simulink model "UPQC_model"  (R2020b)
settings: Solver=FixedStepAuto  StartTime=0.0  StopTime=Tsim  FixedStep=Tsample  MaxStep=Tsample  RelTol=1e-3
values from neighbouring files (symbols this model uses):
  C_parallel_Series = zeros(1,4)    [Netzmodell_Ini_DL.m]    (also in workspace_Ini.mat = [1e-05 1e-05 1e-05 0])
  C_parallel_Shunt = zeros(1,4)    [Netzmodell_Ini_DL.m]    (also in workspace_Ini.mat = [1e-05 1e-05 1e-05 0])
  CC_Ki = 5    [Netzmodell_Ini_DL.m]    (also in workspace_Ini.mat)
  CC_Ki_geg = 5    [Netzmodell_Ini_DL.m]    (also in workspace_Ini.mat)
  CC_Kp = 10    [Netzmodell_Ini_DL.m]    (also in workspace_Ini.mat)
  CC_Kp_geg = 10    [Netzmodell_Ini_DL.m]    (also in workspace_Ini.mat)
  CC_OS =     [workspace_Ini.mat]
  Czk = Szenario.Czk*u    [Netzmodell_Ini_DL.m]    (also in workspace_Ini.mat = 0.003)
  fak_RVC = Szenario.fak_RVC    [Netzmodell_Ini_DL.m]    (also in workspace_Ini.mat = [1 1 1])
  fak_Uns = [1; 1; 1]    [Netzmodell_Ini_DL.m]    (also in workspace_Ini.mat = [1 1 1])
  Flicker_Schaltzeitpunkte_L1 = Schaltzeitpunkte(1,:)    [Netzmodell_Ini_DL.m]    (also in workspace_Ini.mat = 10.5)
  Flicker_Schaltzeitpunkte_L2 = Schaltzeitpunkte(2,:)    [Netzmodell_Ini_DL.m]    (also in workspace_Ini.mat = 10.5)
  Flicker_Schaltzeitpunkte_L3 = Schaltzeitpunkte(3,:)    [Netzmodell_Ini_DL.m]    (also in workspace_Ini.mat = 10.5)
  fs = [f_nom; f_nom; f_nom]    [Netzmodell_Ini_DL.m]    (also in workspace_Ini.mat = [50 50 50])
  fsw = Szenario.fsw*k    [Netzmodell_Ini_DL.m]    (also in workspace_Ini.mat = 20000)
  I_Basis_Ober_L1 = I_Basis_Ober(1)    [Netzmodell_Ini_DL.m]    (also in workspace_Ini.mat = 0)
  I_Basis_Ober_L2 = I_Basis_Ober(2)    [Netzmodell_Ini_DL.m]    (also in workspace_Ini.mat = 0)
  I_Basis_Ober_L3 = I_Basis_Ober(3)    [Netzmodell_Ini_DL.m]    (also in workspace_Ini.mat = 0)
  I_relativ_Ober_L1 = Szenario.I_relativ_Ober_L1    [Netzmodell_Ini_DL.m]    (also in workspace_Ini.mat = [0 100 0 100 100 0 100 100 0 0 0 0 ... (50 elements, 1x50)])
  I_relativ_Ober_L2 = Szenario.I_relativ_Ober_L2    [Netzmodell_Ini_DL.m]    (also in workspace_Ini.mat = [0 100 0 100 100 0 100 100 0 0 0 0 ... (50 elements, 1x50)])
  I_relativ_Ober_L3 = Szenario.I_relativ_Ober_L3    [Netzmodell_Ini_DL.m]    (also in workspace_Ini.mat = [0 100 0 100 100 0 100 100 0 0 0 0 ... (50 elements, 1x50)])
  L_Ausgang_Series = zeros(1,4)    [Netzmodell_Ini_DL.m]    (also in workspace_Ini.mat = [0.00093 0.00093 0.00093 0.00093])
  L_Ausgang_Shunt = zeros(1,4)    [Netzmodell_Ini_DL.m]    (also in workspace_Ini.mat = [0.00093 0.00093 0.00093 0.00093])
  L_Eingang_Series = zeros(1,4)    [Netzmodell_Ini_DL.m]    (also in workspace_Ini.mat = [0.00085 0.00085 0.00085 0.00085])
  L_Eingang_Shunt = zeros(1,4)    [Netzmodell_Ini_DL.m]    (also in workspace_Ini.mat = [0.00085 0.00085 0.00085 0.00085])
  Ls_in = 52.2*u/10    (= 5.22e-06)    [Netzmodell_Ini_DL.m]    (also in workspace_Ini.mat)
  Ltrans = Szenario.Ltrans*m    [Netzmodell_Ini_DL.m]    (also in workspace_Ini.mat = 0.000256)
  OS_off = 6    [Netzmodell_Ini_DL.m]    (also in workspace_Ini.mat)
  OS_on = 1    [Netzmodell_Ini_DL.m]    (also in workspace_Ini.mat)
  Phi_Ober_L1 = Phi_Ober(1)    [Netzmodell_Ini_DL.m]    (also in workspace_Ini.mat = 0)
  Phi_Ober_L2 = Phi_Ober(2)    [Netzmodell_Ini_DL.m]    (also in workspace_Ini.mat = -120)
  Phi_Ober_L3 = Phi_Ober(3)    [Netzmodell_Ini_DL.m]    (also in workspace_Ini.mat = 120)
  Phis = [0; -120; 120]    [Netzmodell_Ini_DL.m]    (also in workspace_Ini.mat = [0 -120 120])
  Pl_Flicker = Pl_Flicker*k    [Netzmodell_Ini_DL.m]    (also in workspace_Ini.mat = [5000 5000 5000])
  Pl_Grund = Szenario.Pl_Grund *k    [Netzmodell_Ini_DL.m]    (also in workspace_Ini.mat = [5 5 5])
  Pl_RVC = Pl_RVC*k    [Netzmodell_Ini_DL.m]    (also in workspace_Ini.mat = [10000 10000 10000])
  Pl_Uns = Pl_Uns*k    [Netzmodell_Ini_DL.m]    (also in workspace_Ini.mat = [25000 10 10])
  Ql_ind_Flicker = Ql_ind_Flicker*k    [Netzmodell_Ini_DL.m]    (also in workspace_Ini.mat = [0 0 0])
  Ql_ind_Grund = Szenario.Ql_ind_Grund*k    [Netzmodell_Ini_DL.m]    (also in workspace_Ini.mat = [0 0 0])
  Ql_ind_RVC = Szenario.Ql_ind_RVC*k    [Netzmodell_Ini_DL.m]    (also in workspace_Ini.mat = [0 0 0])
  Ql_ind_Uns = Ql_ind_Uns*k    [Netzmodell_Ini_DL.m]    (also in workspace_Ini.mat = [0 0 0])
  Ql_kap_Flicker = Ql_kap_Flicker*k    [Netzmodell_Ini_DL.m]    (also in workspace_Ini.mat = [0 0 0])
  Ql_kap_Grund = Szenario.Ql_kap_Grund*k    [Netzmodell_Ini_DL.m]    (also in workspace_Ini.mat = [0 0 0])
  Ql_kap_RVC = Szenario.Ql_kap_RVC*k    [Netzmodell_Ini_DL.m]    (also in workspace_Ini.mat = [0 0 0])
  Ql_kap_Uns = Ql_kap_Uns*k    [Netzmodell_Ini_DL.m]    (also in workspace_Ini.mat = [0 0 0])
  R_Ausgang_Series = zeros(1,4)    [Netzmodell_Ini_DL.m]    (also in workspace_Ini.mat = [0.1 0.1 0.1 0.1])
  R_Ausgang_Shunt = zeros(1,4)    [Netzmodell_Ini_DL.m]    (also in workspace_Ini.mat = [0.1 0.1 0.1 0.1])
  R_Eingang_Series = zeros(1,4)    [Netzmodell_Ini_DL.m]    (also in workspace_Ini.mat = [0.1 0.1 0.1 0.1])
  R_Eingang_Shunt = zeros(1,4)    [Netzmodell_Ini_DL.m]    (also in workspace_Ini.mat = [0.1 0.1 0.1 0.1])
  R_parallel_Series = zeros(1,4)    [Netzmodell_Ini_DL.m]    (also in workspace_Ini.mat = [13 13 13 0])
  R_parallel_Shunt = zeros(1,4)    [Netzmodell_Ini_DL.m]    (also in workspace_Ini.mat = [13 13 13 0])
  R_ZK_Belastung = 20    [Netzmodell_Ini_DL.m]    (also in workspace_Ini.mat)
  Rs_in = 5.2*m/10    (= 0.00052)    [Netzmodell_Ini_DL.m]    (also in workspace_Ini.mat)
  Rtrans = Szenario.Rtrans    [Netzmodell_Ini_DL.m]    (also in workspace_Ini.mat = 0.206)
  RVC_L1_on_off_Zeitpunkte = Szenario.RVC_L1_on_off_Zeitpunkte    [Netzmodell_Ini_DL.m]    (also in workspace_Ini.mat = [10.5 40 10 11 12 13 14 15])
  RVC_L2_on_off_Zeitpunkte = Szenario.RVC_L2_on_off_Zeitpunkte    [Netzmodell_Ini_DL.m]    (also in workspace_Ini.mat = [10.5 40 10 11 12 13 14 15])
  RVC_L3_on_off_Zeitpunkte = Szenario.RVC_L3_on_off_Zeitpunkte    [Netzmodell_Ini_DL.m]    (also in workspace_Ini.mat = [10.5 40 10 11 12 13 14 15])
  RVC_off = 20.5    [Netzmodell_Ini_DL.m]    (also in workspace_Ini.mat)
  RVC_on = 20    [Netzmodell_Ini_DL.m]    (also in workspace_Ini.mat)
  RVC_val = [0.8,0.8,0.8]    [Netzmodell_Ini_DL.m]    (also in workspace_Ini.mat = [0.8 0.8 0.8])
  strans = Szenario.strans    [Netzmodell_Ini_DL.m]    (also in workspace_Ini.mat = 0.25)
  t_breaker_series = tacts    [Netzmodell_Ini_DL.m]    (also in workspace_Ini.mat = 0.5)
  tact = Szenario.tact    [Netzmodell_Ini_DL.m]    (also in workspace_Ini.mat = 0.5)
  tact_OS_Regler = Szenario.tact_OS_Regler    [Netzmodell_Ini_DL.m]    (also in workspace_Ini.mat = 0.5)
  tact_QU = 10    [Netzmodell_Ini_DL.m]    (also in workspace_Ini.mat)
  tacts = Szenario.tacts    [Netzmodell_Ini_DL.m]    (also in workspace_Ini.mat = 0.5)
  Tsample = Szenario.Tsample    [Netzmodell_Ini_DL.m]    (also in workspace_Ini.mat = 5e-06)
  Uns_L1_on_off_Zeitpunkte = Szenario.Uns_L1_on_off_Zeitpunkte    [Netzmodell_Ini_DL.m]    (also in workspace_Ini.mat = [1 6 10 11 12 13 14 15])
  Uns_L2_on_off_Zeitpunkte = Szenario.Uns_L2_on_off_Zeitpunkte    [Netzmodell_Ini_DL.m]    (also in workspace_Ini.mat = [10 30 10 11 12 13 14 15])
  Uns_L3_on_off_Zeitpunkte = Szenario.Uns_L3_on_off_Zeitpunkte    [Netzmodell_Ini_DL.m]    (also in workspace_Ini.mat = [10 30 10 11 12 13 14 15])
  Us = [Us_Amp; Us_Amp; Us_Amp]    [Netzmodell_Ini_DL.m]    (also in workspace_Ini.mat = [326.598632371 326.598632371 326.598632371])
  Us_Amp = sqrt(2)*400/sqrt(3)    [Netzmodell_Ini_DL.m]    (also in workspace_Ini.mat = 326.598632371)
  VC_Ki_gegen = 30    [Netzmodell_Ini_DL.m]    (also in workspace_Ini.mat)
  VC_Ki_gegen_shunt = 15    [Netzmodell_Ini_DL.m]    (also in workspace_Ini.mat)
  VC_Ki_mit = 5    [Netzmodell_Ini_DL.m]    (also in workspace_Ini.mat)
  VC_Kp_gegen = 5    [workspace_Ini.mat]
  VC_Kp_gegen_shunt = 2    [Netzmodell_Ini_DL.m]    (also in workspace_Ini.mat)
  VC_Kp_mit = 10    [Netzmodell_Ini_DL.m]    (also in workspace_Ini.mat)
  VC_ZK_Ki = 5    [Netzmodell_Ini_DL.m]    (also in workspace_Ini.mat)
  VC_ZK_Kp = 0.5    [Netzmodell_Ini_DL.m]    (also in workspace_Ini.mat)
  Vielfache_Ober_L1 = Szenario.Vielfache_Ober_L1    [Netzmodell_Ini_DL.m]    (also in workspace_Ini.mat = [1 2 3 4 5 6 7 8 9 10 11 12 ... (50 elements, 1x50)])
  Vielfache_Ober_L2 = Szenario.Vielfache_Ober_L2    [Netzmodell_Ini_DL.m]    (also in workspace_Ini.mat = [1 2 3 4 5 6 7 8 9 10 11 12 ... (50 elements, 1x50)])
  Vielfache_Ober_L3 = Szenario.Vielfache_Ober_L3    [Netzmodell_Ini_DL.m]    (also in workspace_Ini.mat = [1 2 3 4 5 6 7 8 9 10 11 12 ... (50 elements, 1x50)])
  ZK_Belastung_off = 100    [Netzmodell_Ini_DL.m]    (also in workspace_Ini.mat)
  ZK_Belastung_on = 100    [Netzmodell_Ini_DL.m]    (also in workspace_Ini.mat)
  Zwischenkreisspannung = 700    [Netzmodell_Ini_DL.m]    (also in workspace_Ini.mat)
undefined symbols (not defined in the file or in its folder): LAusgang, RReiheL3
libraries: powerlib x221, powerlib_meascontrol x80, pid_lib x23, eeTransforms x4, eePwmGeneratorTwoLevel x2, dspstat3 x1
(part 4 of 16)

== system UPQC_model/Zwischenkreis_Shunt ==
  Add : Sum
  C Zwischenkreis1 : powerlib/Elements/Series RLC Branch  LConnTagsString=__new0  RConnTagsString=__new0  BranchType=C  Resistance=RReiheL3  Inductance=2.4e-3  SetiL0=off  InitialCurrent=0  Capacitance=C_Zwischenkreis*2  Setx0=off  InitialVoltage=350  Measurements=None
  C Zwischenkreis2 : powerlib/Elements/Series RLC Branch  LConnTagsString=__new0  RConnTagsString=__new0  BranchType=C  Resistance=RReiheL3  Inductance=2.4e-3  SetiL0=off  InitialCurrent=0  Capacitance=C_Zwischenkreis*2  Setx0=off  InitialVoltage=350  Measurements=None
  Ground : powerlib/Elements/Ground  Commented=on  LConnTagsString=a
  I DC 1 : powerlib/Measurements/Current Measurement  PhasorSimulation=off  OutputType=Complex  PSBequivalent=0
  I DC 2 : powerlib/Measurements/Current Measurement  PhasorSimulation=off  OutputType=Complex  PSBequivalent=0
  I DC 3 : powerlib/Measurements/Current Measurement  PhasorSimulation=off  OutputType=Complex  PSBequivalent=0
  I DC in : powerlib/Measurements/Current Measurement  PhasorSimulation=off  OutputType=Complex  PSBequivalent=0
  Series RLC Branch2 : powerlib/Elements/Series RLC Branch  LConnTagsString=__new0  RConnTagsString=__new0  BranchType=R  Resistance=40e3  Inductance=2.4e-3  SetiL0=off  InitialCurrent=0  Capacitance=C_Zwischenkreis  Setx0=off  InitialVoltage=0  Measurements=None
  Shunt_Zwischenkreise_I_Scope : Scope  NumInputPorts=4
  U DC: : powerlib/Measurements/Voltage Measurement  PhasorSimulation=off  OutputType=Complex  PSBequivalent=0
  DC+ out : PMIOPort  Side=Right
  DC- out : PMIOPort  Port=2  Side=Right
  DC+ in : PMIOPort  Port=3  Side=Left
  DC- in : PMIOPort  Port=4  Side=Left
  Neutral Connection : PMIOPort  Tag=PMCPort  Port=5  Side=Left
  U DC Zwischenkreis : Outport
  I DC Zwischenkreis out : Outport  Port=2
  I DC Zwischenkreis in : Outport  Port=3
  wires:
  U DC:/1 -> U DC Zwischenkreis/1
  I DC in/1 -> I DC Zwischenkreis out/1
  I DC 1/1 -> Add/1, I DC Zwischenkreis in/1, Shunt_Zwischenkreise_I_Scope/1
  I DC 2/1 -> Add/2, Shunt_Zwischenkreise_I_Scope/2
  Add/1 -> Shunt_Zwischenkreise_I_Scope/3
  I DC 3/1 -> Shunt_Zwischenkreise_I_Scope/4
  connections:
  C Zwischenkreis2/RConn1 -- Neutral Connection/RConn1 -- Ground/LConn1 -- C Zwischenkreis1/LConn1
  Series RLC Branch2/LConn1 -- I DC 3/RConn1
  I DC 2/LConn1 -- DC- in/RConn1
  I DC 1/LConn1 -- DC+ in/RConn1
  I DC in/RConn1 -- DC+ out/RConn1
  C Zwischenkreis1/RConn1 -- U DC:/LConn2 -- DC- out/RConn1 -- Series RLC Branch2/RConn1 -- I DC 2/RConn1
  U DC:/LConn1 -- I DC 3/LConn1 -- C Zwischenkreis2/LConn1 -- I DC 1/RConn1 -- I DC in/LConn1

== system UPQC_model/Messsignale/A ==
  Vabc : Inport
  I : Inport  Port=2
  Constant : Constant  Value=Us_Amp
  Demux : Demux  Outputs=3
  Divide{1..5} (5 alike) : Product  Inputs=*/
  Gain : Gain  Gain=100
  Gain1 : Gain  Gain=100
  Gain2 : Gain  Gain=0.001
  Mux : Mux  Inputs=2
  Mux1 : Mux  Inputs=2
  Mux2 : Mux  Inputs=3
  Power : powerlib_meascontrol/Measurements/Power  Freq=50  Vinit=[1, 0]  Iinit=[1, 0]  Ts=0
  Sequence Analyzer : powerlib_meascontrol/Measurements/Sequence Analyzer  Freq=f_nom  n=1  seq=Positive Negative Zero  InInit=[1, 0]  Ts=0
      settings: SourceProductBaseCode=PS
  +-0 normiert : Outport
  PQ : Outport  Port=2
  kU2,kU0 : Outport  Port=3
  Phase +-0 : Outport  Port=4
  wires:
  [Normierung] -> Divide3/2, Divide2/2, Divide1/2
  Divide1/1 -> Mux2/1, Divide5/2, Divide4/2  "+,A"
  Demux/1 -> Divide1/1
  I/1 -> Power/2
  Vabc/1 -> Power/1, Sequence Analyzer/1
  Divide3/1 -> Mux2/3, Divide5/1  "0,A"
  Demux/3 -> Divide3/1
  Constant/1 -> [Normierung]
  Power/2 -> Mux1/2  "Q, A"
  Demux/2 -> Divide2/1
  Divide2/1 -> Mux2/2, Divide4/1  "-,A"
  Sequence Analyzer/2 -> Phase +-0/1
  Power/1 -> Mux1/1  "P, A"
  Divide4/1 -> Gain/1  "kU2"
  Divide5/1 -> Gain1/1  "kU0"
  Sequence Analyzer/1 -> Demux/1
  Mux/1 -> kU2,kU0/1  "kU2, kU0"
  Mux1/1 -> Gain2/1  "PQ, A"
  Mux2/1 -> +-0 normiert/1  "+-0, A"
  Gain/1 -> Mux/1
  Gain1/1 -> Mux/2
  Gain2/1 -> PQ/1

== system UPQC_model/Messsignale/A1 ==
  Vabc : Inport
  I : Inport  Port=2
  Constant : Constant  Value=Us_Amp
  Demux : Demux  Outputs=3
  Divide{1..5} (5 alike) : Product  Inputs=*/
  Gain : Gain  Gain=100
  Gain1 : Gain  Gain=100
  Gain2 : Gain  Gain=0.001
  Mux : Mux  Inputs=2
  Mux1 : Mux  Inputs=2
  Mux2 : Mux  Inputs=3
  Power : powerlib_meascontrol/Measurements/Power  Freq=50  Vinit=[1, 0]  Iinit=[1, 0]  Ts=0
  Sequence Analyzer : powerlib_meascontrol/Measurements/Sequence Analyzer  Freq=f_nom  n=1  seq=Positive Negative Zero  InInit=[1, 0]  Ts=0
      settings: SourceProductBaseCode=PS
  +-0 normiert : Outport
  PQ : Outport  Port=2
  "kU2, kU0" : Outport  Port=3
  Phase +-0 : Outport  Port=4
  wires:
  [Normierung] -> Divide3/2, Divide2/2, Divide1/2
  Divide1/1 -> Mux2/1, Divide5/2, Divide4/2  "+,A"
  Demux/1 -> Divide1/1
  I/1 -> Power/2
  Vabc/1 -> Power/1, Sequence Analyzer/1
  Divide3/1 -> Mux2/3, Divide5/1  "0,A"
  Demux/3 -> Divide3/1
  Constant/1 -> [Normierung]
  Power/2 -> Mux1/2  "Q, A"
  Demux/2 -> Divide2/1
  Divide2/1 -> Mux2/2, Divide4/1  "-,A"
  Sequence Analyzer/2 -> Phase +-0/1
  Power/1 -> Mux1/1  "P, A"
  Divide4/1 -> Gain/1  "kU2"
  Divide5/1 -> Gain1/1  "kU0"
  Sequence Analyzer/1 -> Demux/1
  Mux/1 -> "kU2, kU0"/1  "kU2, kU0"
  Mux1/1 -> Gain2/1  "PQ, A"
  Mux2/1 -> +-0 normiert/1  "+-0, A"
  Gain/1 -> Mux/1
  Gain1/1 -> Mux/2
  Gain2/1 -> PQ/1

== system UPQC_model/Messsignale/Bneu ==
  Vabc : Inport
  I : Inport  Port=2
  Constant : Constant  Value=Us_Amp
  Demux : Demux  Outputs=3
  Divide{1..5} (5 alike) : Product  Inputs=*/
  Gain : Gain  Gain=100
  Gain1 : Gain  Gain=100
  Gain2 : Gain  Gain=0.001
  Mux : Mux  Inputs=2
  Mux1 : Mux  Inputs=2
  Mux2 : Mux  Inputs=3
  Power : powerlib_meascontrol/Measurements/Power  Freq=50  Vinit=[1, 0]  Iinit=[1, 0]  Ts=0
  Sequence Analyzer : powerlib_meascontrol/Measurements/Sequence Analyzer  Freq=f_nom  n=1  seq=Positive Negative Zero  InInit=[1, 0]  Ts=0
      settings: SourceProductBaseCode=PS
  +-0 normiert : Outport
  PQ : Outport  Port=2
  "kU2, kU0" : Outport  Port=3
  Phase +-0 : Outport  Port=4
  wires:
  [Normierung] -> Divide3/2, Divide2/2, Divide1/2
  Divide1/1 -> Mux2/1, Divide5/2, Divide4/2  "+,A"
  Demux/1 -> Divide1/1
  I/1 -> Power/2
  Vabc/1 -> Power/1, Sequence Analyzer/1
  Divide3/1 -> Mux2/3, Divide5/1  "0,A"
  Demux/3 -> Divide3/1
  Constant/1 -> [Normierung]
  Power/2 -> Mux1/2  "Q, A"
  Demux/2 -> Divide2/1
  Divide2/1 -> Mux2/2, Divide4/1  "-,A"
  Sequence Analyzer/2 -> Phase +-0/1
  Power/1 -> Mux1/1  "P, A"
  Divide4/1 -> Gain/1  "kU2"
  Divide5/1 -> Gain1/1  "kU0"
  Sequence Analyzer/1 -> Demux/1
  Mux/1 -> "kU2, kU0"/1  "kU2, kU0"
  Mux1/1 -> Gain2/1  "PQ, A"
  Mux2/1 -> +-0 normiert/1  "+-0, A"
  Gain/1 -> Mux/1
  Gain1/1 -> Mux/2
  Gain2/1 -> PQ/1

== system UPQC_model/Oberschwingung Last/50 Times Input ==
  Constant : Constant  Value=0
  Mux : Mux  Inputs=50
  Out1 : Outport
  wires:
  Mux/1 -> Out1/1
  Constant/1 -> Mux/50, Mux/49, Mux/48, Mux/47, Mux/46, Mux/45, Mux/44, Mux/43, Mux/42, Mux/41, Mux/40, Mux/39, Mux/38, Mux/37, Mux/36, Mux/35, Mux/34, Mux/33, Mux/32, Mux/31, Mux/30, Mux/29, Mux/28, Mux/27, Mux/26, Mux/25, Mux/24, Mux/23, Mux/22, Mux/21, Mux/20, Mux/19, Mux/18, Mux/17, Mux/16, Mux/15, Mux/14, Mux/13, Mux/12, Mux/11, Mux/10, Mux/9, Mux/8, Mux/7, Mux/6, Mux/5, Mux/4, Mux/3, Mux/2, Mux/1

== system UPQC_model/Oberschwingung Last/Subsystem1 ==
  Constant : Constant  Value=-120
  Mux : Mux  Inputs=50
  Out1 : Outport
  wires:
  Mux/1 -> Out1/1
  Constant/1 -> Mux/50, Mux/49, Mux/48, Mux/47, Mux/46, Mux/45, Mux/44, Mux/43, Mux/42, Mux/41, Mux/40, Mux/39, Mux/38, Mux/37, Mux/36, Mux/35, Mux/34, Mux/33, Mux/32, Mux/31, Mux/30, Mux/29, Mux/28, Mux/27, Mux/26, Mux/25, Mux/24, Mux/23, Mux/22, Mux/21, Mux/20, Mux/19, Mux/18, Mux/17, Mux/16, Mux/15, Mux/14, Mux/13, Mux/12, Mux/11, Mux/10, Mux/9, Mux/8, Mux/7, Mux/6, Mux/5, Mux/4, Mux/3, Mux/2, Mux/1

== system UPQC_model/Oberschwingung Last/Subsystem2 ==
  Constant : Constant  Value=120
  Mux : Mux  Inputs=50
  Out1 : Outport
  wires:
  Constant/1 -> Mux/1, Mux/2, Mux/3, Mux/4, Mux/5, Mux/6, Mux/7, Mux/8, Mux/9, Mux/10, Mux/11, Mux/12, Mux/13, Mux/14, Mux/15, Mux/16, Mux/17, Mux/18, Mux/19, Mux/20, Mux/21, Mux/22, Mux/23, Mux/24, Mux/25, Mux/26, Mux/27, Mux/28, Mux/29, Mux/30, Mux/31, Mux/32, Mux/33, Mux/34, Mux/35, Mux/36, Mux/37, Mux/38, Mux/39, Mux/40, Mux/41, Mux/42, Mux/43, Mux/44, Mux/45, Mux/46, Mux/47, Mux/48, Mux/49, Mux/50
  Mux/1 -> Out1/1

== system UPQC_model/Series UPQC/Serienkompensator ==
  note: OUTPUT
  note: INPUT
  note: --------------------------------------------------------------------------------
  note: --------------------------------------------------------------------------------
  note: --------------------------------------------------------------------------------
  note: --------------------------------------------------------------------------------
  note: SETPOINT GENERATION
  note: ARCHIV
  note: SPANNUNGSREGELUNG
  note: REFERENZSPANNUNG LAST
  note: ISTSPANNUNG LAST
  enable : Inport
  PLL : Inport  Port=2
  VSC-Strom : Inport  Port=3
  PCC-Spg : Inport  Port=4
  Bus Selector : BusSelector  OutputSignals=phipll
  Bus Selector1 : BusSelector  OutputSignals=udqp1_f,udqg1_f
  Gegensystem : Subsystem
  Mitsystem : Subsystem
  Setpoints Series : Scope  NumInputPorts=2
  Step : Step  Time=tacts  SampleTime=0
  Subsystem : Subsystem
  Subsystem3 : Subsystem
  Subsystem5 : Subsystem
  Udq_Series_C : Subsystem
  dq+ Soll VSC Series : Scope
  dq- Last : Scope
  dq- Soll VSC Series : Scope
  sp : Outport
  wires:
  PCC-Spg/1 -> [ext_spg]
  VSC-Strom/1 -> [int_strom]
  [setpoints] -> sp/1
  enable/1 -> [enable]
  [ext_spg] -> Setpoints Series/1  "C_Netzspannung_abc"
  [udq0gegREF] -> Gegensystem/1(udq0ref)
  [udq0geg] -> Gegensystem/2(udq0)
  [phipll] -> Subsystem3/2(phiPLL)
  Subsystem3/1(sp) -> [setpoints], Setpoints Series/2  "Setpoints_Series"
  Subsystem/1(udq0ref) -> [udq0mitREF]
  Subsystem5/1(udq0ref) -> [udq0gegREF]
  PLL/1 -> Bus Selector/1
  Bus Selector/1 -> [phipll]  "<phipll>"
  [udq0mitREF] -> Mitsystem/1(udq0ref)
  [udq0mit] -> Mitsystem/2(udq0)
  Step/1 -> Mitsystem/Enable, Gegensystem/Enable
  [udq0mitsp] -> Subsystem3/1(upos)
  Mitsystem/1(udq0*) -> dq+ Soll VSC Series/1, [udq0mitsp]  "udq0*+"
  Gegensystem/1(udq0*) -> dq- Soll VSC Series/1, [udq0gegsp]  "udq0*-"
  [phipll] -> Udq_Series_C/2(In1)  "pll"
  Udq_Series_C/1(Out5) -> Bus Selector1/1
  Bus Selector1/1 -> [udq0mit]  "<udqp1_f>"
  Bus Selector1/2 -> dq- Last/1, [udq0geg]  "<udqg1_f>"
  [ext_spg] -> Udq_Series_C/1(In2)
  [udq0gegsp] -> Subsystem3/3(uneg)

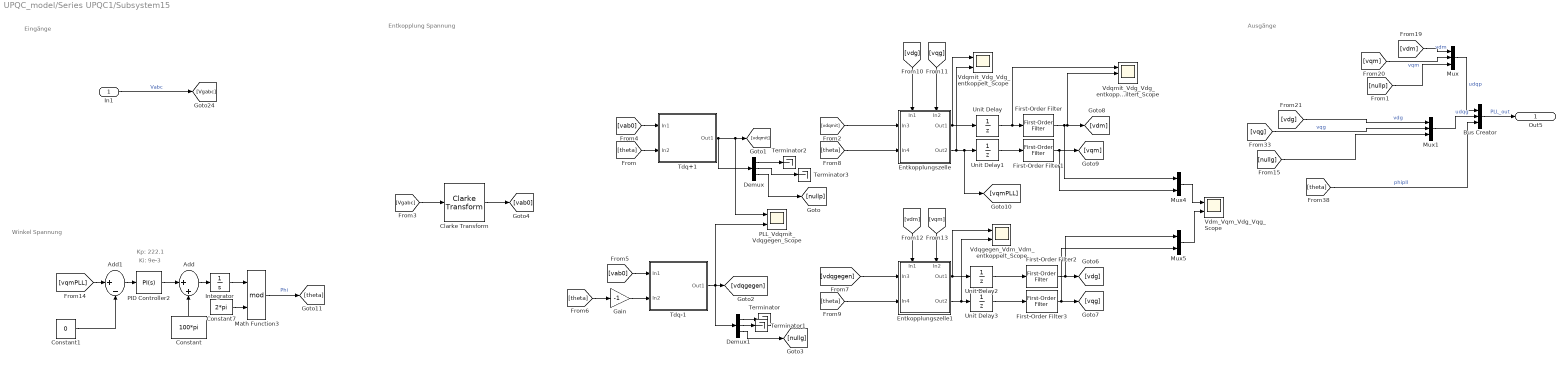
== system UPQC_model/Series UPQC1/Subsystem15 ==
  note: Ki: 9e-3
  note: Kp: 222.1
  note: Winkel Spannung
  note: Ausgänge
  note: Eingänge
  note: Entkopplung Spannung
  In1 : Inport
  Add : Sum  Inputs=|++
  Add1 : Sum  Inputs=|+-
  Bus Creator : BusCreator  Inputs=3
  Clarke Transform : eeTransforms/Clarke Transform  PowerInvariant=off
      settings: SourceProductBaseCode=PS
  Constant : Constant  Value=100*pi
  Constant1 : Constant  Value=0
  Constant7 : Constant  Value=2*pi
  Demux : Demux  Outputs=3
  Demux1 : Demux  Outputs=3
  Entkopplungszelle : Subsystem
      settings: PortSchema="{\"entries\":[{\"content\":{\"sides\":[{\"content\":{\"connectorIds\":[\"In1\",\"In2\"]},\"type\":\"ConnectorPlacement.EquallySpacedRectSide\",\"uuid\":\"e8e24803-2fc0-483c-82f9-6ee33f65ebd9\"},{\"content\":{\"connectorIds\":[\"Out1\",\"Out2\"],\"side\":\"RIGHT\"},\"type\":\"ConnectorPlacement.EquallySpacedRectSide\",\"uuid\":\"e11e5831-ab5e-42bb-bd0b-63825273f403\"},{\"content\":{\"connectorIds\":[\"In3\",\"In4\"],\"side\":\"TOP\"},\"type\":\"ConnectorPlacement.EquallySpacedRectSide\",\"uuid\":\"2b39bd07-2b6e-4e89-bb54-1321cea2c793\"},{\"content\":{\"connectorIds\":[],\"side\":\"HIDDEN\"},\"type\":\"ConnectorPlacement.EquallySpacedRectSide\",\"uuid\":\"a99c5943-5af0-4d11-8875-695bd24f17f4\"}]},\"type\":\"ConnectorPlacement.EquallySpacedConnector\",\"uuid\":\"a2a714db-f067-4e0e-8919-f68d1dab84ba\"}],\"packageUris\":[\"http://schema.mathworks.com/mf0/Connector/R2020b\"],\"version\":\"1.0\"}"
  Entkopplungszelle1 : Subsystem
      settings: PortSchema="{\"entries\":[{\"content\":{\"sides\":[{\"content\":{\"connectorIds\":[\"In1\",\"In2\"]},\"type\":\"ConnectorPlacement.EquallySpacedRectSide\",\"uuid\":\"e8e24803-2fc0-483c-82f9-6ee33f65ebd9\"},{\"content\":{\"connectorIds\":[\"Out1\",\"Out2\"],\"side\":\"RIGHT\"},\"type\":\"ConnectorPlacement.EquallySpacedRectSide\",\"uuid\":\"e11e5831-ab5e-42bb-bd0b-63825273f403\"},{\"content\":{\"connectorIds\":[\"In3\",\"In4\"],\"side\":\"TOP\"},\"type\":\"ConnectorPlacement.EquallySpacedRectSide\",\"uuid\":\"2b39bd07-2b6e-4e89-bb54-1321cea2c793\"},{\"content\":{\"connectorIds\":[],\"side\":\"HIDDEN\"},\"type\":\"ConnectorPlacement.EquallySpacedRectSide\",\"uuid\":\"a99c5943-5af0-4d11-8875-695bd24f17f4\"}]},\"type\":\"ConnectorPlacement.EquallySpacedConnector\",\"uuid\":\"a2a714db-f067-4e0e-8919-f68d1dab84ba\"}],\"packageUris\":[\"http://schema.mathworks.com/mf0/Connector/R2020b\"],\"version\":\"1.0\"}"
  First-Order Filter{,1..3} (4 alike) : powerlib_meascontrol/Filters/First-Order Filter  FilterType=Lowpass  Tc=1/(2*pi*50/sqrt(2))  Ts=0  Initialize=off  Vac_Init=[0, 0, 60]  Vdc_Init=0  PlotResponse=off  FreqRange="[0,  30,  1]"
  Gain : Gain  Gain=-1
  Integrator : Integrator
  Math Function3 : Math  Operator=mod  SignedPower=on  SaturateOnIntegerOverflow=on
  Mux : Mux  Inputs=3
  Mux1 : Mux  Inputs=3
  Mux4 : Mux  Inputs=2
  Mux5 : Mux  Inputs=2
  PID Controller2 : pid_lib/PID Controller  Controller=PI  Form=Parallel  TimeDomain=Continuous-time  UseExternalTs=off  SampleTime=-1  IntegratorMethod=Forward Euler  FilterMethod=Forward Euler  ControllerParametersSource=internal  P=222.1  I=9e-3  D=0  UseFilter=on  N=100  TunerSelectOption=Transfer Function Based (PID Tuner App)  InitialConditionSource=internal  InitialConditionForIntegrator=0  InitialConditionForFilter=0  DifferentiatorICPrevScaledInput=0  ExternalReset=none  TrackingMode=off  Kt=1  LimitOutput=off  SatLimitsSource=internal  UpperSaturationLimit=inf  LowerSaturationLimit=-inf  LinearizeAsGain=on  AntiWindupMode=none  Kb=1  POutMin=[]  POutMax=[]  IOutMin=[]  IOutMax=[]  DOutMin=[]  DOutMax=[]  NOutMin=[]  NOutMax=[]  SumOutMin=[]  SumOutMax=[]  SaturationOutMin=[]  SaturationOutMax=[]  PParamMin=[]  PParamMax=[]  IParamMin=[]  IParamMax=[]  DParamMin=[]  DParamMax=[]  NParamMin=[]  NParamMax=[]  KbParamMin=[]  KbParamMax=[]  KtParamMin=[]  KtParamMax=[]  KbOutMin=[]  KbOutMax=[]  KtOutMin=[]  KtOutMax=[]  IntegratorOutMin=[]  IntegratorOutMax=[]  FilterOutMin=[]  FilterOutMax=[]  SumI1OutMin=[]  SumI1OutMax=[]  SumI2OutMin=[]  SumI2OutMax=[]  SumI3OutMin=[]  SumI3OutMax=[]  SumI4OutMin=[]  SumI4OutMax=[]  SumDOutMin=[]  SumDOutMax=[]  DifferentiatorOutMin=[]  DifferentiatorOutMax=[]  FilterDiffOutCoefMin=[]  FilterDiffOutCoefMax=[]  ReciprocalOutMin=[]  ReciprocalOutMax=[]  SumDenOutMin=[]  SumDenOutMax=[]  SumNumOutMin=[]  SumNumOutMax=[]  DivideOutMin=[]  DivideOutMax=[]  UdiffTsProdOutMin=[]  UdiffTsProdOutMax=[]  NTsProdOutMin=[]  NTsProdOutMax=[]  UintegralTsProdOutMin=[]  UintegralTsProdOutMax=[]  UngainTsProdOutMin=[]  UngainTsProdOutMax=[]  IntegratorContinuousStateAttributes=''  IntegratorStateMustResolveToSignalObject=off  IntegratorRTWStateStorageClass=Auto  FilterContinuousStateAttributes=''  FilterStateMustResolveToSignalObject=off  FilterRTWStateStorageClass=Auto  ParallelPVariant=InternalParameters  IdealPVariant=Disabled  IVariant=InternalParameters  DVariant=Disabled  IntegratorVariant=Continuous  SatVariant=Disabled  AWVariant=Passthrough  PCopyVariant=Disabled  TRVariant=Disabled  FdbkBlocksVariant=Forward  IdealPFdbkVariant=Disabled  SatFdbkVariant=Disabled  DerivativeFilterVariant=Disabled  NVariant=Disabled  NCopyVariant=Disabled_SignalSpec  FilterICVariant=Disabled  IntegratorICVariant=InternalICs  ExternalResetVariant=Disabled  TRSumVariant=Passthrough  SumFdbkVariant=Disabled  SumVariant=Sum_PI  TsampFilterVariant=InternalTs  TsampNgainVariant=Passthrough  TsampIntegralVariant=Passthrough  ExternalSaturationOutDataTypeStr=Inherit: Same as second input
  PLL_Vdqmit_Vdqgegen_Scope : Scope  NumInputPorts=2
  Tdq+1 : Subsystem
  Tdq-1 : Subsystem
  Terminator{,1..3} (4 alike) : Terminator
  Unit Delay{,1..3} (4 alike) : UnitDelay  SampleTime=-1  HasFrameUpgradeWarning=on
  Vdm_Vqm_Vdg_Vqg_Scope : Scope  NumInputPorts=2
  Vdqgegen_Vdm_Vdm_entkoppelt_Scope : Scope  NumInputPorts=2
  Vdqmit_Vdg_Vdg_entkoppelt_Scope : Scope  NumInputPorts=2
  Vdqmit_Vdg_Vdg_entkoppelt_gefiltert_Scope : Scope  NumInputPorts=3
  Out5 : Outport
  wires:
  [theta] -> Entkopplungszelle/2(In4)
  Clarke Transform/1 -> [vab0]
  [vdqmit] -> Entkopplungszelle/1(In3)
  [vqm] -> Entkopplungszelle1/4(In2)
  Entkopplungszelle1/2(Out2) -> Vdqgegen_Vdm_Vdm_entkoppelt_Scope/2, Unit Delay3/1
  Constant/1 -> Add/2
  Tdq-1/1(Out1) -> Demux1/1, [vdqgegen], PLL_Vdqmit_Vdqgegen_Scope/2
  [vdg] -> Entkopplungszelle/3(In1)
  Unit Delay/1 -> Vdqmit_Vdg_Vdg_entkoppelt_gefiltert_Scope/1, First-Order Filter/1
  Entkopplungszelle/2(Out2) -> Vdqmit_Vdg_Vdg_entkoppelt_Scope/2, [vqmPLL], Unit Delay1/1
  Constant1/1 -> Add1/2
  [vqmPLL] -> Add1/1
  Integrator/1 -> Math Function3/1
  [theta] -> Gain/1
  Gain/1 -> Tdq-1/2(In2)
  [vdm] -> Entkopplungszelle1/3(In1)
  [vqg] -> Entkopplungszelle/4(In2)
  Add/1 -> Integrator/1
  Unit Delay3/1 -> First-Order Filter3/1
  First-Order Filter/1 -> Mux4/1, [vdm], Vdqmit_Vdg_Vdg_entkoppelt_gefiltert_Scope/2
  [theta] -> Tdq+1/2(In2)
  Constant7/1 -> Math Function3/2
  [vab0] -> Tdq-1/1(In1)
  PID Controller2/1 -> Add/1
  Unit Delay1/1 -> First-Order Filter1/1
  Add1/1 -> PID Controller2/1
  [theta] -> Entkopplungszelle1/2(In4)
  [vdqgegen] -> Entkopplungszelle1/1(In3)
  In1/1 -> [Vgabc]  "Vabc"
  [vdg] -> Mux1/1  "vdg"
  [vqg] -> Mux1/2  "vqg"
  [theta] -> Bus Creator/3  "phipll"
  Math Function3/1 -> [theta]  "Phi"
  [vab0] -> Tdq+1/1(In1)
  Entkopplungszelle/1(Out1) -> Vdqmit_Vdg_Vdg_entkoppelt_Scope/1, Unit Delay/1
  Entkopplungszelle1/1(Out1) -> Vdqgegen_Vdm_Vdm_entkoppelt_Scope/1, Unit Delay2/1
  [Vgabc] -> Clarke Transform/1
  Bus Creator/1 -> Out5/1  "PLL_out"
  Tdq+1/1(Out1) -> Demux/1, PLL_Vdqmit_Vdqgegen_Scope/1, [vdqmit]
  Demux1/1 -> Terminator/1
  Demux1/2 -> Terminator1/1
  Demux/1 -> Terminator2/1
  Demux/2 -> Terminator3/1
  Demux/3 -> [nullp]
  Demux1/3 -> [nullg]
  [vdm] -> Mux/1  "vdm"
  [vqm] -> Mux/2  "vqm"
  [nullp] -> Mux/3
  Mux/1 -> Bus Creator/1  "udqp"
  [nullg] -> Mux1/3
  Mux1/1 -> Bus Creator/2  "udqg"
  Unit Delay2/1 -> First-Order Filter2/1
  Mux5/1 -> Vdm_Vqm_Vdg_Vqg_Scope/2
  Mux4/1 -> Vdm_Vqm_Vdg_Vqg_Scope/1
  First-Order Filter1/1 -> [vqm], Mux4/2
  First-Order Filter2/1 -> [vdg], Mux5/1
  First-Order Filter3/1 -> [vqg], Mux5/2

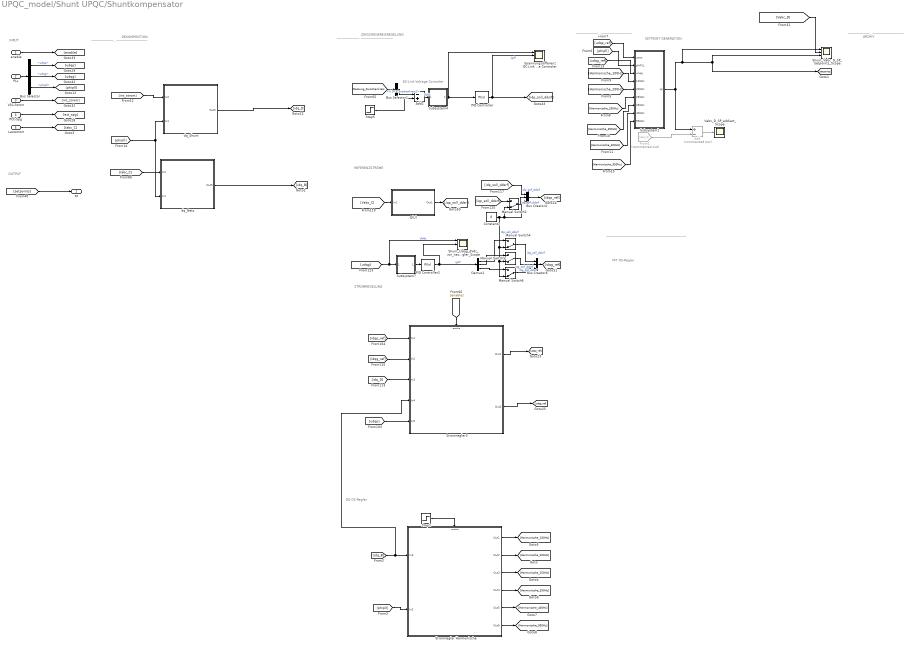
== system UPQC_model/Shunt UPQC/Shuntkompensator ==
  note: DC-Link Voltage Controler
  note: --------------------------------------------------------------------------------
  note: DEKOMPOSITION
  note: REFERENZSTRÖME
  note: STROMREGELUNG
  note: ARCHIV
  note: OUTPUT
  note: INPUT
  note: SETPOINT GENERATION
  note: --------------------------------------------------------------------------------
  note: --------------------------------------------------------------------------------
  note: --------------------------------------------------------------------------------
  note: --------------------------------------------------------------------------------
  note: FFT OS-Regler
  note: DQ OS-Regler
  note: ZWISCHENKREISREGELUNG
  enable : Inport
  PLL : Inport  Port=2
  VSC-Strom : Inport  Port=3
  PCC-Spg : Inport  Port=4
  Laststrom : Inport  Port=5
  Add : Sum  Commented=on  Inputs=+-
  Add2 : Sum  Inputs=-+
  Bus Creator4 : BusCreator  Inputs=3
  Bus Creator6 : BusCreator  Inputs=3
  Bus Selector : BusSelector  OutputSignals=udqp,udqg,phipll
  Bus Selector1 : BusSelector  OutputSignals=U DC Zwischenkreis1
  Constant1 : Constant  Value=0
  Demux1 : Demux  Outputs=3
  From1 : From  Commented=on  GotoTag=Vabc_D  TagVisibility=global
  Manual Switch{2,4..6} (4 alike) : ManualSwitch  CurrentSetting=0
  PID Controller : pid_lib/PID Controller  Controller=PI  Form=Parallel  TimeDomain=Continuous-time  UseExternalTs=off  SampleTime=-1  IntegratorMethod=Forward Euler  FilterMethod=Forward Euler  ControllerParametersSource=internal  P=VC_ZK_Kp  I=VC_ZK_Ki  D=0  UseFilter=on  N=100  TunerSelectOption=Transfer Function Based (PID Tuner App)  InitialConditionSource=internal  InitialConditionForIntegrator=0  InitialConditionForFilter=0  DifferentiatorICPrevScaledInput=0  ExternalReset=none  TrackingMode=off  Kt=1  LimitOutput=off  SatLimitsSource=internal  UpperSaturationLimit=5  LowerSaturationLimit=-5  LinearizeAsGain=on  AntiWindupMode=none  Kb=1  POutMin=[]  POutMax=[]  IOutMin=[]  IOutMax=[]  DOutMin=[]  DOutMax=[]  NOutMin=[]  NOutMax=[]  SumOutMin=[]  SumOutMax=[]  SaturationOutMin=[]  SaturationOutMax=[]  PParamMin=[]  PParamMax=[]  IParamMin=[]  IParamMax=[]  DParamMin=[]  DParamMax=[]  NParamMin=[]  NParamMax=[]  KbParamMin=[]  KbParamMax=[]  KtParamMin=[]  KtParamMax=[]  KbOutMin=[]  KbOutMax=[]  KtOutMin=[]  KtOutMax=[]  IntegratorOutMin=[]  IntegratorOutMax=[]  FilterOutMin=[]  FilterOutMax=[]  SumI1OutMin=[]  SumI1OutMax=[]  SumI2OutMin=[]  SumI2OutMax=[]  SumI3OutMin=[]  SumI3OutMax=[]  SumI4OutMin=[]  SumI4OutMax=[]  SumDOutMin=[]  SumDOutMax=[]  DifferentiatorOutMin=[]  DifferentiatorOutMax=[]  FilterDiffOutCoefMin=[]  FilterDiffOutCoefMax=[]  ReciprocalOutMin=[]  ReciprocalOutMax=[]  SumDenOutMin=[]  SumDenOutMax=[]  SumNumOutMin=[]  SumNumOutMax=[]  DivideOutMin=[]  DivideOutMax=[]  UdiffTsProdOutMin=[]  UdiffTsProdOutMax=[]  NTsProdOutMin=[]  NTsProdOutMax=[]  UintegralTsProdOutMin=[]  UintegralTsProdOutMax=[]  UngainTsProdOutMin=[]  UngainTsProdOutMax=[]  IntegratorContinuousStateAttributes=''  IntegratorStateMustResolveToSignalObject=off  IntegratorRTWStateStorageClass=Auto  FilterContinuousStateAttributes=''  FilterStateMustResolveToSignalObject=off  FilterRTWStateStorageClass=Auto  ParallelPVariant=InternalParameters  IdealPVariant=Disabled  IVariant=InternalParameters  DVariant=Disabled  IntegratorVariant=Continuous  SatVariant=Disabled  AWVariant=Passthrough  PCopyVariant=Disabled  TRVariant=Disabled  FdbkBlocksVariant=Forward  IdealPFdbkVariant=Disabled  SatFdbkVariant=Disabled  DerivativeFilterVariant=Disabled  NVariant=Disabled  NCopyVariant=Disabled_SignalSpec  FilterICVariant=Disabled  IntegratorICVariant=InternalICs  ExternalResetVariant=Disabled  TRSumVariant=Passthrough  SumFdbkVariant=Disabled  SumVariant=Sum_PI  TsampFilterVariant=InternalTs  TsampNgainVariant=Passthrough  TsampIntegralVariant=Passthrough  ExternalSaturationOutDataTypeStr=Inherit: Same as second input
  PID Controller2 : pid_lib/PID Controller  Controller=PI  Form=Parallel  TimeDomain=Continuous-time  UseExternalTs=off  SampleTime=-1  IntegratorMethod=Forward Euler  FilterMethod=Forward Euler  ControllerParametersSource=internal  P=VC_Kp_gegen_shunt  I=VC_Ki_gegen_shunt  D=0  UseFilter=on  N=100  TunerSelectOption=Transfer Function Based (PID Tuner App)  InitialConditionSource=internal  InitialConditionForIntegrator=0  InitialConditionForFilter=0  DifferentiatorICPrevScaledInput=0  ExternalReset=none  TrackingMode=off  Kt=1  LimitOutput=off  SatLimitsSource=internal  UpperSaturationLimit=5  LowerSaturationLimit=-5  LinearizeAsGain=on  AntiWindupMode=none  Kb=1  POutMin=[]  POutMax=[]  IOutMin=[]  IOutMax=[]  DOutMin=[]  DOutMax=[]  NOutMin=[]  NOutMax=[]  SumOutMin=[]  SumOutMax=[]  SaturationOutMin=[]  SaturationOutMax=[]  PParamMin=[]  PParamMax=[]  IParamMin=[]  IParamMax=[]  DParamMin=[]  DParamMax=[]  NParamMin=[]  NParamMax=[]  KbParamMin=[]  KbParamMax=[]  KtParamMin=[]  KtParamMax=[]  KbOutMin=[]  KbOutMax=[]  KtOutMin=[]  KtOutMax=[]  IntegratorOutMin=[]  IntegratorOutMax=[]  FilterOutMin=[]  FilterOutMax=[]  SumI1OutMin=[]  SumI1OutMax=[]  SumI2OutMin=[]  SumI2OutMax=[]  SumI3OutMin=[]  SumI3OutMax=[]  SumI4OutMin=[]  SumI4OutMax=[]  SumDOutMin=[]  SumDOutMax=[]  DifferentiatorOutMin=[]  DifferentiatorOutMax=[]  FilterDiffOutCoefMin=[]  FilterDiffOutCoefMax=[]  ReciprocalOutMin=[]  ReciprocalOutMax=[]  SumDenOutMin=[]  SumDenOutMax=[]  SumNumOutMin=[]  SumNumOutMax=[]  DivideOutMin=[]  DivideOutMax=[]  UdiffTsProdOutMin=[]  UdiffTsProdOutMax=[]  NTsProdOutMin=[]  NTsProdOutMax=[]  UintegralTsProdOutMin=[]  UintegralTsProdOutMax=[]  UngainTsProdOutMin=[]  UngainTsProdOutMax=[]  IntegratorContinuousStateAttributes=''  IntegratorStateMustResolveToSignalObject=off  IntegratorRTWStateStorageClass=Auto  FilterContinuousStateAttributes=''  FilterStateMustResolveToSignalObject=off  FilterRTWStateStorageClass=Auto  ParallelPVariant=InternalParameters  IdealPVariant=Disabled  IVariant=InternalParameters  DVariant=Disabled  IntegratorVariant=Continuous  SatVariant=Disabled  AWVariant=Passthrough  PCopyVariant=Disabled  TRVariant=Disabled  FdbkBlocksVariant=Forward  IdealPFdbkVariant=Disabled  SatFdbkVariant=Disabled  DerivativeFilterVariant=Disabled  NVariant=Disabled  NCopyVariant=Disabled_SignalSpec  FilterICVariant=Disabled  IntegratorICVariant=InternalICs  ExternalResetVariant=Disabled  TRSumVariant=Passthrough  SumFdbkVariant=Disabled  SumVariant=Sum_PI  TsampFilterVariant=InternalTs  TsampNgainVariant=Passthrough  TsampIntegralVariant=Passthrough  ExternalSaturationOutDataTypeStr=Inherit: Same as second input
  Q(U) : Subsystem
  Shunt_Udqg_dVdc_vor_nach_PIRegler_Scope : Scope  NumInputPorts=3
  Shunt_Vabc_D_SP_Setpoints_Scope : Scope  NumInputPorts=3
  Spannungsdifferenz DC Link Voltage Controler : Scope  NumInputPorts=3
  Step1 : Step  Time=tact_OS_Regler  SampleTime=0
  Step5 : Step  Time=100  Before=Zwischenkreisspannung  After=Zwischenkreisspannung+0  SampleTime=0
  Stromregler Harmonische : Subsystem
  Stromregler3 : Subsystem
  Subsystem1 : Subsystem
  Subsystem4 : Subsystem
  Subsystem7 : Subsystem
  Vabc_D_SP_addiert_Scope : Scope
  dq_Netz : Subsystem
  dq_Shunt : Subsystem
  sp : Outport
  wires:
  [int_strom] -> dq_Shunt/1(In2)
  enable/1 -> [enable]
  [setpoints] -> sp/1
  PCC-Spg/1 -> [ext_spg]
  Laststrom/1 -> [Iabc_C]
  VSC-Strom/1 -> [int_strom]
  PLL/1 -> Bus Selector/1
  [phipll] -> dq_Netz/2(In1), dq_Shunt/2(In1)
  [Iabc_C] -> dq_Netz/1(In2)
  Bus Selector/1 -> [udqp]  "<udqp>"
  Bus Selector/2 -> [udqg]  "<udqg>"
  Subsystem1/1(sp) -> Add/1, Shunt_Vabc_D_SP_Setpoints_Scope/3, [setpoints], Shunt_Vabc_D_SP_Setpoints_Scope/1
  [Messung_Zwischenkreis] -> Bus Selector1/1
  Bus Selector1/1 -> Add2/1  "<U DC Zwischenkreis1>"
  PID Controller/1 -> Spannungsdifferenz DC Link Voltage Controler/2, [idp_soll_ddsrf]  "igd*"
  Step5/1 -> Add2/2
  Stromregler3/2(Out2) -> [udqg_ref]
  Stromregler3/1(Out1) -> [udqp_ref]
  [enable] -> Stromregler3/Enable
  [idqp_ref] -> Stromregler3/1(In1)
  [idqg_ref] -> Stromregler3/2(In2)
  Bus Creator4/1 -> [idqp_ref]
  [idp_soll_ddsrf] -> Bus Creator4/1  "idp_soll_ddsrf"
  [idq_D] -> Stromregler3/3(In3)
  [Vabc_C] -> Q(U)/1(In1)
  Q(U)/1(Out1) -> [iqp_soll_ddsrf]
  Add2/1 -> Subsystem4/1(dVdc)  "dVdc"
  [udqg] -> Shunt_Udqg_dVdc_vor_nach_PIRegler_Scope/1, Subsystem7/1(dVdc)  "dVdc"
  PID Controller2/1 -> Demux1/1, Shunt_Udqg_dVdc_vor_nach_PIRegler_Scope/2  "igd*"
  Subsystem7/1(Gatesignale_(6)) -> PID Controller2/1
  [udqp] -> Stromregler3/5(In5)
  Bus Creator6/1 -> [idqg_ref]
  Constant1/1 -> Manual Switch2/2, Bus Creator4/3, Manual Switch4/2, Manual Switch6/2, Manual Switch5/2  "i0p_soll_ddsrf"
  Manual Switch2/1 -> Bus Creator4/2  "iqp_soll_ddsrf"
  [iqp_soll_ddsrf] -> Manual Switch2/1
  Demux1/1 -> Manual Switch4/1
  Demux1/2 -> Manual Switch5/1
  Demux1/3 -> Manual Switch6/1
  Manual Switch4/1 -> Bus Creator6/1  "idg_soll_ddsrf"
  Manual Switch5/1 -> Bus Creator6/2  "iqg_soll_ddsrf"
  Manual Switch6/1 -> Bus Creator6/3  "i0g_soll_ddsrf"
  dq_Shunt/1(Out5) -> [idq_D]
  dq_Netz/1(Out5) -> [idq_B]
  From1/1 -> Add/2
  Add/1 -> Vabc_D_SP_addiert_Scope/1
  [idq_B] -> Stromregler Harmonische/1(In3), Stromregler3/4(In4)
  Step1/1 -> Stromregler Harmonische/Enable
  [phipll] -> Stromregler Harmonische/2(In2)
  Bus Selector/3 -> [phipll]  "<phipll>"
  Stromregler Harmonische/2(Out2) -> [Harmonische_200Hz]
  Stromregler Harmonische/5(Out5) -> [Harmonische_400Hz]
  [Vabc_D] -> Shunt_Vabc_D_SP_Setpoints_Scope/2
  Subsystem4/1(Gatesignale_(6)) -> PID Controller/1, Spannungsdifferenz DC Link Voltage Controler/1
  [Harmonische_400Hz] -> Subsystem1/8(400Hz)
  [Harmonische_200Hz] -> Subsystem1/5(200Hz)
  [Harmonische_100Hz] -> Subsystem1/4(100Hz)
  [Harmonische_950Hz] -> Subsystem1/9(950Hz)
  [Harmonische_350Hz] -> Subsystem1/7(350Hz)
  [phipll] -> Subsystem1/2(phiPLL)
  [Harmonische_250Hz] -> Subsystem1/6(250Hz)
  [udqg_ref] -> Subsystem1/3(uneg)
  [udqp_ref] -> Subsystem1/1(upos)
  Stromregler Harmonische/1(Out1) -> [Harmonische_100Hz]
  Stromregler Harmonische/3(Out3) -> [Harmonische_250Hz]
  Stromregler Harmonische/4(Out4) -> [Harmonische_350Hz]
  Stromregler Harmonische/6(Out6) -> [Harmonische_950Hz]

== system UPQC_model/VSC_Series_U/Subsystem4 ==
  dVdc : Inport
  Constant1 : Constant  Value=0
  Step1 : Step  Time=tacts  SampleTime=0
  Switch : Switch  Criteria=u2 > Threshold
  Gatesignale_(6) : Outport
  wires:
  Switch/1 -> Gatesignale_(6)/1
  dVdc/1 -> Switch/1
  Constant1/1 -> Switch/3
  Step1/1 -> Switch/2

== system UPQC_model/VSC_Shunt_U/Subsystem4 ==
  dVdc : Inport
  Constant1 : Constant  Value=0
  Step1 : Step  Time=tact  SampleTime=0
  Switch : Switch  Criteria=u2 > Threshold
  Gatesignale_(6) : Outport
  wires:
  Switch/1 -> Gatesignale_(6)/1
  dVdc/1 -> Switch/1
  Constant1/1 -> Switch/3
  Step1/1 -> Switch/2

== system UPQC_model/Series UPQC/Serienkompensator/Gegensystem ==
  udq0ref : Inport
  udq0 : Inport  Port=2
  Enable : EnablePort
  Add : Sum
  Add1 : Sum
  Constant : Constant
  Constant1 : Constant
  Constant5 : Constant  Value=0
  Gain : Gain  Gain=10
  Gain1 : Gain
  Gain2 : Gain  Commented=on  Gain=-1
  Gain3 : Gain
  Gain6 : Gain  Gain=-1
  Integrator : Integrator
  Mux6 : Mux  Inputs=3
  PID Controller2 : pid_lib/PID Controller  Controller=PI  Form=Parallel  TimeDomain=Continuous-time  UseExternalTs=off  SampleTime=-1  IntegratorMethod=Forward Euler  FilterMethod=Forward Euler  ControllerParametersSource=internal  P=VC_Kp_gegen  I=VC_Ki_gegen  D=0  UseFilter=on  N=100  TunerSelectOption=Transfer Function Based (PID Tuner App)  InitialConditionSource=internal  InitialConditionForIntegrator=0  InitialConditionForFilter=0  DifferentiatorICPrevScaledInput=0  ExternalReset=none  TrackingMode=off  Kt=1  LimitOutput=off  SatLimitsSource=internal  UpperSaturationLimit=inf  LowerSaturationLimit=-inf  LinearizeAsGain=on  AntiWindupMode=none  Kb=1  POutMin=[]  POutMax=[]  IOutMin=[]  IOutMax=[]  DOutMin=[]  DOutMax=[]  NOutMin=[]  NOutMax=[]  SumOutMin=[]  SumOutMax=[]  SaturationOutMin=[]  SaturationOutMax=[]  PParamMin=[]  PParamMax=[]  IParamMin=[]  IParamMax=[]  DParamMin=[]  DParamMax=[]  NParamMin=[]  NParamMax=[]  KbParamMin=[]  KbParamMax=[]  KtParamMin=[]  KtParamMax=[]  KbOutMin=[]  KbOutMax=[]  KtOutMin=[]  KtOutMax=[]  IntegratorOutMin=[]  IntegratorOutMax=[]  FilterOutMin=[]  FilterOutMax=[]  SumI1OutMin=[]  SumI1OutMax=[]  SumI2OutMin=[]  SumI2OutMax=[]  SumI3OutMin=[]  SumI3OutMax=[]  SumI4OutMin=[]  SumI4OutMax=[]  SumDOutMin=[]  SumDOutMax=[]  DifferentiatorOutMin=[]  DifferentiatorOutMax=[]  FilterDiffOutCoefMin=[]  FilterDiffOutCoefMax=[]  ReciprocalOutMin=[]  ReciprocalOutMax=[]  SumDenOutMin=[]  SumDenOutMax=[]  SumNumOutMin=[]  SumNumOutMax=[]  DivideOutMin=[]  DivideOutMax=[]  UdiffTsProdOutMin=[]  UdiffTsProdOutMax=[]  NTsProdOutMin=[]  NTsProdOutMax=[]  UintegralTsProdOutMin=[]  UintegralTsProdOutMax=[]  UngainTsProdOutMin=[]  UngainTsProdOutMax=[]  IntegratorContinuousStateAttributes=''  IntegratorStateMustResolveToSignalObject=off  IntegratorRTWStateStorageClass=Auto  FilterContinuousStateAttributes=''  FilterStateMustResolveToSignalObject=off  FilterRTWStateStorageClass=Auto  ParallelPVariant=InternalParameters  IdealPVariant=Disabled  IVariant=InternalParameters  DVariant=Disabled  IntegratorVariant=Continuous  SatVariant=Disabled  AWVariant=Passthrough  PCopyVariant=Disabled  TRVariant=Disabled  FdbkBlocksVariant=Forward  IdealPFdbkVariant=Disabled  SatFdbkVariant=Disabled  DerivativeFilterVariant=Disabled  NVariant=Disabled  NCopyVariant=Disabled_SignalSpec  FilterICVariant=Disabled  IntegratorICVariant=InternalICs  ExternalResetVariant=Disabled  TRSumVariant=Passthrough  SumFdbkVariant=Disabled  SumVariant=Sum_PI  TsampFilterVariant=InternalTs  TsampNgainVariant=Passthrough  TsampIntegralVariant=Passthrough  ExternalSaturationOutDataTypeStr=Inherit: Same as second input
  PID Controller3 : pid_lib/PID Controller  Controller=PI  Form=Parallel  TimeDomain=Continuous-time  UseExternalTs=off  SampleTime=-1  IntegratorMethod=Forward Euler  FilterMethod=Forward Euler  ControllerParametersSource=internal  P=VC_Kp_gegen  I=VC_Ki_gegen  D=0  UseFilter=on  N=100  TunerSelectOption=Transfer Function Based (PID Tuner App)  InitialConditionSource=internal  InitialConditionForIntegrator=0  InitialConditionForFilter=0  DifferentiatorICPrevScaledInput=0  ExternalReset=none  TrackingMode=off  Kt=1  LimitOutput=off  SatLimitsSource=internal  UpperSaturationLimit=inf  LowerSaturationLimit=-inf  LinearizeAsGain=on  AntiWindupMode=none  Kb=1  POutMin=[]  POutMax=[]  IOutMin=[]  IOutMax=[]  DOutMin=[]  DOutMax=[]  NOutMin=[]  NOutMax=[]  SumOutMin=[]  SumOutMax=[]  SaturationOutMin=[]  SaturationOutMax=[]  PParamMin=[]  PParamMax=[]  IParamMin=[]  IParamMax=[]  DParamMin=[]  DParamMax=[]  NParamMin=[]  NParamMax=[]  KbParamMin=[]  KbParamMax=[]  KtParamMin=[]  KtParamMax=[]  KbOutMin=[]  KbOutMax=[]  KtOutMin=[]  KtOutMax=[]  IntegratorOutMin=[]  IntegratorOutMax=[]  FilterOutMin=[]  FilterOutMax=[]  SumI1OutMin=[]  SumI1OutMax=[]  SumI2OutMin=[]  SumI2OutMax=[]  SumI3OutMin=[]  SumI3OutMax=[]  SumI4OutMin=[]  SumI4OutMax=[]  SumDOutMin=[]  SumDOutMax=[]  DifferentiatorOutMin=[]  DifferentiatorOutMax=[]  FilterDiffOutCoefMin=[]  FilterDiffOutCoefMax=[]  ReciprocalOutMin=[]  ReciprocalOutMax=[]  SumDenOutMin=[]  SumDenOutMax=[]  SumNumOutMin=[]  SumNumOutMax=[]  DivideOutMin=[]  DivideOutMax=[]  UdiffTsProdOutMin=[]  UdiffTsProdOutMax=[]  NTsProdOutMin=[]  NTsProdOutMax=[]  UintegralTsProdOutMin=[]  UintegralTsProdOutMax=[]  UngainTsProdOutMin=[]  UngainTsProdOutMax=[]  IntegratorContinuousStateAttributes=''  IntegratorStateMustResolveToSignalObject=off  IntegratorRTWStateStorageClass=Auto  FilterContinuousStateAttributes=''  FilterStateMustResolveToSignalObject=off  FilterRTWStateStorageClass=Auto  ParallelPVariant=InternalParameters  IdealPVariant=Disabled  IVariant=InternalParameters  DVariant=Disabled  IntegratorVariant=Continuous  SatVariant=Disabled  AWVariant=Passthrough  PCopyVariant=Disabled  TRVariant=Disabled  FdbkBlocksVariant=Forward  IdealPFdbkVariant=Disabled  SatFdbkVariant=Disabled  DerivativeFilterVariant=Disabled  NVariant=Disabled  NCopyVariant=Disabled_SignalSpec  FilterICVariant=Disabled  IntegratorICVariant=InternalICs  ExternalResetVariant=Disabled  TRSumVariant=Passthrough  SumFdbkVariant=Disabled  SumVariant=Sum_PI  TsampFilterVariant=InternalTs  TsampNgainVariant=Passthrough  TsampIntegralVariant=Passthrough  ExternalSaturationOutDataTypeStr=Inherit: Same as second input
  Product1 : Product
  Product2 : Product
  Relational Operator : RelationalOperator  OutDataTypeStr=boolean  RndMeth=Simplest
  Selector5 : Selector  InputPortWidth=2  IndexOptions=Index vector (dialog)  Indices=[1]  OutputSizes=1
  Selector6 : Selector  InputPortWidth=2  IndexOptions=Index vector (dialog)  Indices=[1]  OutputSizes=1
  Selector7 : Selector  InputPortWidth=2  IndexOptions=Index vector (dialog)  Indices=[2]  OutputSizes=1
  Selector8 : Selector  InputPortWidth=2  IndexOptions=Index vector (dialog)  Indices=[2]  OutputSizes=1
  Series_Kompensator_Gegensys_udq0_kreuz_d_vor_nach_PI_Scope : Scope  NumInputPorts=3
  Series_Kompensator_Gegensys_udq0_kreuz_q_vor_nach_PI_Scope : Scope  NumInputPorts=3
  Subtract2 : Sum  Inputs=+-
  Subtract3 : Sum  Inputs=+-
  Switch : Switch  Threshold=1
  wLqm->dm : Gain  Commented=on  Gain=100*pi*(L_Eingang_Shunt(1,1) +L_Ausgang_Shunt(1,1))
  wLqm->dm1 : Gain  Commented=on  Gain=100*pi*(L_Eingang_Shunt(1,1) +L_Ausgang_Shunt(1,1))
  udq0* : Outport
  wires:
  Constant5/1 -> Mux6/3
  Selector5/1 -> Series_Kompensator_Gegensys_udq0_kreuz_d_vor_nach_PI_Scope/1, wLqm->dm/1, Subtract2/2
  Selector7/1 -> wLqm->dm1/1, Series_Kompensator_Gegensys_udq0_kreuz_q_vor_nach_PI_Scope/1, Subtract3/2
  Selector8/1 -> Subtract3/1
  Selector6/1 -> Subtract2/1
  Mux6/1 -> Gain6/1
  [udq0ref] -> Selector8/1
  [udq0ref] -> Selector6/1
  udq0ref/1 -> [udq0ref]
  udq0/1 -> [udq0]
  Add1/1 -> Gain3/1
  Subtract2/1 -> Product1/1, Series_Kompensator_Gegensys_udq0_kreuz_d_vor_nach_PI_Scope/2
  wLqm->dm/1 -> Gain2/1
  PID Controller3/1 -> Series_Kompensator_Gegensys_udq0_kreuz_d_vor_nach_PI_Scope/3, Add/1
  Add/1 -> Gain1/1
  wLqm->dm1/1 -> Add/2
  PID Controller2/1 -> Add1/2, Series_Kompensator_Gegensys_udq0_kreuz_q_vor_nach_PI_Scope/3
  Gain2/1 -> Add1/1
  [udq0] -> Selector5/1  "idqp1_f"
  [udq0] -> Selector7/1  "idqp1_f"
  Gain1/1 -> Mux6/1
  Gain3/1 -> Mux6/2
  Gain6/1 -> udq0*/1
  Constant1/1 -> Integrator/1
  Constant/1 -> Switch/1, Relational Operator/2
  Relational Operator/1 -> Switch/2
  Integrator/1 -> Gain/1
  Gain/1 -> Switch/3, Relational Operator/1
  Product1/1 -> PID Controller3/1
  Switch/1 -> Product2/1, Product1/2
  Subtract3/1 -> Series_Kompensator_Gegensys_udq0_kreuz_q_vor_nach_PI_Scope/2, Product2/2
  Product2/1 -> PID Controller2/1
